simulink subsystem "ct_control_ref_subsys"  (R2022b)
settings: Solver=VariableStepAuto  StartTime=0.0  StopTime=10.0  RelTol=1e-3
undefined symbols (not defined in the file): ct_ctrl_param, param_robot
settings Model: Creator=emu  LastModifiedBy=emu

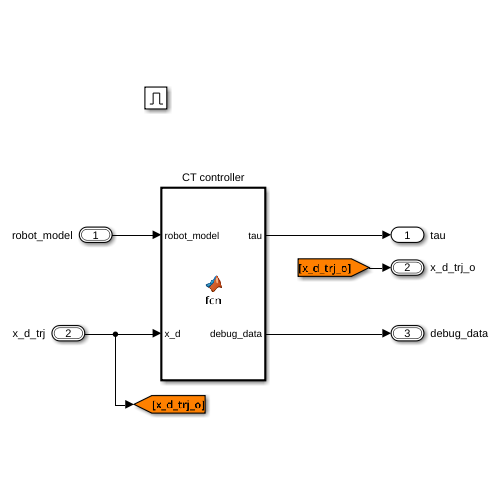
[thumbnail: Simulink's stored preview of the top-level diagram]
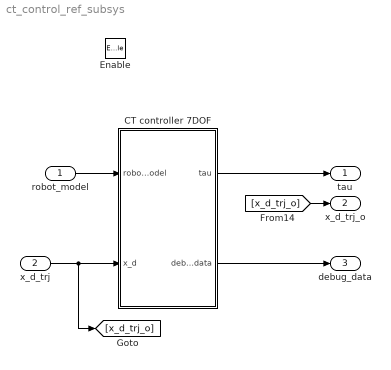
== system ct_control_ref_subsys ==
  robot_model : Inport  OutDataTypeStr=Bus: robot_model
  x_d_trj : Inport  Port=2  OutDataTypeStr=Bus: x_d
  Enable : EnablePort
  CT controller 7DOF : MATLAB Function  TreatAsAtomicUnit=on
  tau : Outport
  x_d_trj_o : Outport  Port=2  OutDataTypeStr=Bus: x_d
  debug_data : Outport  Port=3  OutDataTypeStr=Bus: debug_data_bus
  wires:
  robot_model/1 -> CT controller 7DOF/1(robot_model)
  CT controller 7DOF/1(tau) -> tau/1
  CT controller 7DOF/2(debug_data) -> debug_data/1
  x_d_trj/1 -> [x_d_trj_o], CT controller 7DOF/2(x_d)
  [x_d_trj_o] -> x_d_trj_o/1

== matlab function ct_control_ref_subsys/CT controller 7DOF ==
  settings: updateMethod=DISCRETE  sampleTime=param_global.Ta
  data: tau output; robot_model input Bus: robot_model; x_d input Bus: x_d; ct_ctrl_param parameter; debug_data output Bus: debug_data_bus; param_robot parameter
function [tau, debug_data] = fcn(robot_model, x_d, ct_ctrl_param, param_robot)

% Parameters
q = robot_model.q;      % generalized coordinates
q_p = robot_model.q_p;  % time derivative of generalized coordinates
q_pp = robot_model.q_pp;
M = robot_model.M;      % inertia matrix
%C = robot_model.C;      % coriolis matrix
%g = robot_model.g;      % gravitational forces
C_rnea = robot_model.C_rnea; % C_rnea(q, q_p) = C(q, q_p)q_p + g(q) = n(q, q_p)

J = robot_model.J;      % geometric jacobian to end-effector

J_p = robot_model.J_p;  % time derivative of geometric jacobian to end-effector
H = robot_model.H;


% Control parameters
% kartesisch
Kp1 = ct_ctrl_param.Kp1;
Kd1 = ct_ctrl_param.Kd1;

% nullspace-controller
D_n = ct_ctrl_param.D_n;
K_n = ct_ctrl_param.K_n;
q_n = ct_ctrl_param.q_n;

% Current Pose of Endeffector
x_p = J*q_p;
x_pp = J*q_pp + J_p*q_p;

p = H(1:3,4);
R = H(1:3,1:3);
p_p  = x_p(1:3);
omega_e = x_p(4:6); % Drehwinkelgeschwindigkeit des Endeffektors
% omega_e_p = x_pp(4:6);

% Desired Trajectory
p_d    = x_d.p_d;
p_d_p  = x_d.p_d_p;
p_d_pp = x_d.p_d_pp;
q_d = x_d.q_d;
R_d = x_d.R_d;
omega_d = x_d.omega_d;
omega_d_p = x_d.omega_d_p;

% Errors
RR = R*R_d';
q_err   = rotation2quaternion(RR); %q_err   = rotm2quat_v3(R*R_d');

q_e = quat_mult(q_d, q_err);
%q_e = rotation2quaternion(R);

x_err   = [p-p_d;      q_err(2:4)];   % Error as quaternion
x_err_p = [p_p-p_d_p;  omega_e-omega_d];
x_d_pp  = [p_d_pp;     omega_d_p];


% CT control lawC*q_p + g
%% Cartesian Endeffector Pose
%x_err = [ p- x_d.p_d; q_err(2:4)'];   % Error as quaternion
%x_err_p = [p_p - x_d.p_d_p; omega_e - x_d.omega_d];
%v = J\(x_d_pp  - Kd1*x_err_p - Kp1*x_err - J_p*q_p);
%v = inv(J(1:2,1:2))*(x_d_pp(1:2)  - Kd1(1:2,1:2)*x_err_p(1:2) - Kp1(1:2,1:2)*x_err(1:2) - J_p(1:2,1:2)*q_p);
% sing_method = ct_ctrl_param.mode;

% if(sing_method == 0)
%     J_pinv = pinv(J);
% %elseif(sing_method == 1) % add +k*E
% else
%     k = ct_ctrl_param.k;
%     J_pinv = (J'*J + k*eye(7))\J';
% end
%{
elseif(sing_method == 2) % add +lambda*E
    w_bar_N = ct_ctrl_param.w_bar_N;
    W_E = ct_ctrl_param.W_E;
    e = x_err;
    E_k = 1/2*e' * W_E * e;
    W_N = diag(E_k + w_bar_N);

    [U, S, V] = svd(sqrt(W_E)*J);

    %H_k = V*(S^2 + W_N)*V'; % geht nur wenn alle w_n gleich sind
    H_k = V*(S^2)*V' + W_N;
    J_pinv = H_k\J';

    %J_pinv = (J'*W_E*J + W_N)\J';
    %v = J_pinv*(p_d_pp - Kd1*(p_p - p_d_p) - Kp1*(p - p_d) - J_p*q_p);
    
    %J_new = (J'*W_E*J + W_N);
    %v = J_new\(p_d_pp - Kd1*(p_p - p_d_p) - Kp1*(p - p_d) - J_p*q_p);

else % remove small singular values
    % Perform SVD
    [U, S, V] = svd(J);
    
    % Set a threshold for small singular values
    epsilon = ct_ctrl_param.eps; % Adjust epsilon as needed
    
    % Threshold small singular values in S
    S_new = diag(max(diag(S), epsilon));  % Creates a diagonal matrix with thresholded values
    
    % Reconstruct the matrix with modified singular values
    J_new = U * S_new * V';
    J_pinv = pinv(J_new);
    %v = J_new\(p_d_pp - Kd1*(p_p - p_d_p) - Kp1*(p - p_d) - J_p*q_p);
end
%}

v = J\(x_d_pp - Kd1*x_err_p - Kp1*x_err - J_p*q_p);

%%{
% (V1) NL spring
f_kn = nl_spring_force(q, ct_ctrl_param, param_robot);

% alter nullraumregler
v_n = (-D_n * q_p - K_n * (q - q_n) + f_kn); %(3.43) Pritzi, PD LAW

% neu mit gradientenbasierten nullraumregler
% m_iiwa = sqrt(det(J_iiwa*J_iiwa'));
% J_part_prod = reshape(J_part_iiwa, 6,7,7).*repmat(J_iiwa_inv', 1, 1, 7);
% m_iiwa_diff = m_iiwa*reshape(sum(J_part_prod, [1 2]), 7,1);
% v_n = K_n_grad*[0;0;m_iiwa_diff] - D_n*q_p - K_n * (q - q_n) + f_kn; %(3.57a) TimBoye & Pritzi

% only necessary for 7DOF case.
Minv = M\eye(7);
Minv = 0.5*(Minv + transpose(Minv));
lambdaM = (J*Minv*transpose(J))\eye(6);
lambdaM = 0.5*(lambdaM + transpose(lambdaM));
J_pinv = Minv * transpose(J) * lambdaM; % rechte dynamische gewichtete Pseuodinverse (siehe grundlagen der Robotik) (744 altes skript)


v_nullspace = (eye(7) - J'*J_pinv') * v_n;
tau_n = M * v_nullspace; %(3.41) Pritzi

% tau = M*v + C*q_p + g + tau_n;
tau = M*v + C_rnea + tau_n;
%}
%tau = M*v + C_rnea;

%% DEBUG
debug_data.p    = p;
debug_data.p_p  = p_p;
debug_data.p_pp = x_pp(1:3);
debug_data.Phi  = rotm2rpy(R);
debug_data.Phi_p = zeros(3,1);
debug_data.Phi_pp = zeros(3,1);
debug_data.q       = q_e;
debug_data.omega   = omega_e;
debug_data.omega_p = x_pp(4:6);
debug_data.p_err = x_err(1:3);
debug_data.p_p_err = x_err_p(1:3);
debug_data.p_pp_err = x_pp(1:3) - x_d_pp(1:3);
debug_data.q_err = q_err;
debug_data.omega_err = x_err_p(4:6);
debug_data.omega_p_err = x_pp(4:6) - x_d_pp(4:6);
